simulink model "full_passive_1"  (Simulink 4.00)
settings: Solver=ode45  StartTime=0.0  StopTime=10  RelTol=1e-3
libraries: simulink3 x2
settings Model: LastModifiedBy=administrator

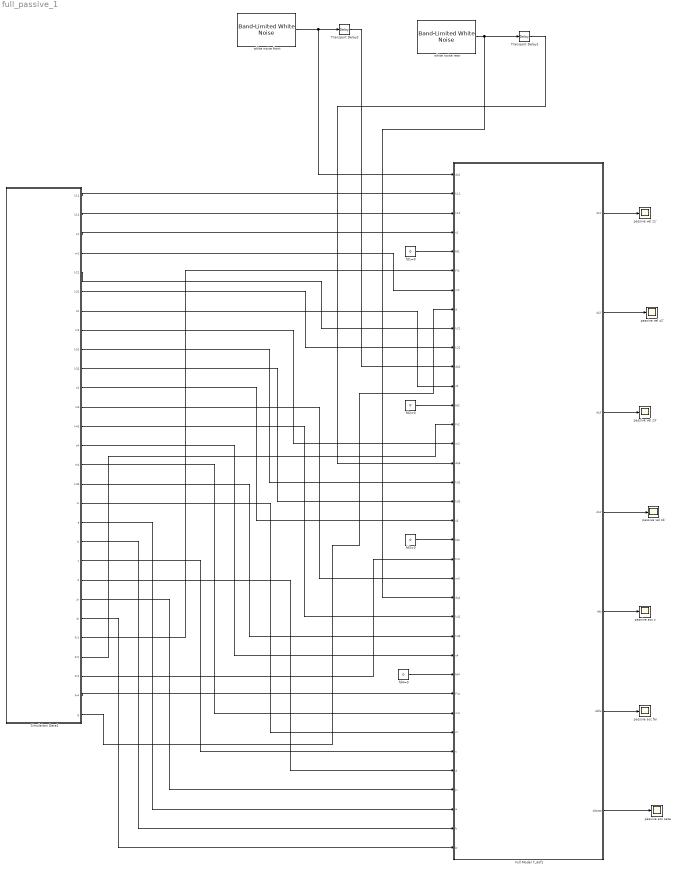
== system full_passive_1 ==
  " white noise front" : simulink3/Sources/Band-Limited White Noise  Cov=[256*10^-6]  Ts=0.01  seed=[23341]
  " white noise rear" : simulink3/Sources/Band-Limited White Noise  Cov=[256*10^-6]  Ts=0.01  seed=[23341]
  Full Model 7_dof1 : Subsystem
      settings: RTWFcnNameOpts=Auto  RTWFileNameOpts=Auto
  Simulaiton Data1 : Subsystem
      settings: RTWFcnNameOpts=Auto  RTWFileNameOpts=Auto
  Transport Delay1 : TransportDelay  DelayTime=1  InitialInput=0  BufferSize=1024  PadeOrder=0
  Transport Delay2 : TransportDelay  DelayTime=1  InitialInput=0  BufferSize=1024  PadeOrder=0
  fd1=0 : Constant  Value=0
  fd2=0 : Constant  Value=0
  fd3=0 : Constant  Value=0
  fd4=0 : Constant  Value=0
  passive acc fai : Scope
      settings: TimeRange=auto  YMin=-5  YMax=5  SaveToWorkspace=off  SaveName=ScopeData  LimitDataPoints=on  MaxDataPoints=5000
  passive acc seta : Scope
      settings: TimeRange=auto  YMin=-5  YMax=5  SaveToWorkspace=off  SaveName=ScopeData14  LimitDataPoints=on  MaxDataPoints=5000
  passive acc z : Scope
      settings: TimeRange=auto  YMin=-5  YMax=5  SaveToWorkspace=off  LimitDataPoints=on  MaxDataPoints=5000
  passive vel z1' : Scope
      settings: TimeRange=auto  YMin=-5  YMax=5  SaveToWorkspace=off  SaveName=ScopeData5  LimitDataPoints=on  MaxDataPoints=5000
  passive vel z2' : Scope
      settings: TimeRange=auto  YMin=-5  YMax=5  SaveToWorkspace=off  SaveName=ScopeData4  LimitDataPoints=on  MaxDataPoints=5000
  passive vel z3' : Scope
      settings: TimeRange=auto  YMin=-5  YMax=5  SaveToWorkspace=off  SaveName=ScopeData3  LimitDataPoints=on  MaxDataPoints=5000
  passive vel z4' : Scope
      settings: TimeRange=auto  YMin=-5  YMax=5  SaveToWorkspace=off  SaveName=ScopeData2  LimitDataPoints=on  MaxDataPoints=5000
  wires:
  " white noise front"/1 -> Transport Delay2/1, Full Model 7_dof1/1(dq1)
  Full Model 7_dof1/7(ddseta) -> passive acc seta/1
  Full Model 7_dof1/6(ddfai) -> passive acc fai/1
  Full Model 7_dof1/5(ddz) -> passive acc z/1
  Full Model 7_dof1/4(dz4') -> passive vel z4'/1
  Full Model 7_dof1/3(dz3') -> passive vel z3'/1
  Full Model 7_dof1/2(dz2') -> passive vel z2'/1
  Full Model 7_dof1/1(dz1') -> passive vel z1'/1
  Transport Delay2/1 -> Full Model 7_dof1/11(dq2)
  " white noise rear"/1 -> Transport Delay1/1, Full Model 7_dof1/23(dq4)
  Transport Delay1/1 -> Full Model 7_dof1/16(dq3)
  fd1=0/1 -> Full Model 7_dof1/5(fd1)
  fd2=0/1 -> Full Model 7_dof1/13(fd2)
  fd3=0/1 -> Full Model 7_dof1/20(fd3)
  fd4=0/1 -> Full Model 7_dof1/27(fd4)
  Simulaiton Data1/1("k11 ") -> Full Model 7_dof1/2(k11)
  Simulaiton Data1/2(k12) -> Full Model 7_dof1/3(k12)
  Simulaiton Data1/3(c1) -> Full Model 7_dof1/4(c1)
  Simulaiton Data1/4(m1) -> Full Model 7_dof1/7(m1)
  Simulaiton Data1/5(k21) -> Full Model 7_dof1/9(k21)
  Simulaiton Data1/6(k22) -> Full Model 7_dof1/10(k22)
  Simulaiton Data1/7(c2) -> Full Model 7_dof1/12(c2)
  Simulaiton Data1/8(m2) -> Full Model 7_dof1/15(m2)
  Simulaiton Data1/9(k31) -> Full Model 7_dof1/17(k31)
  Simulaiton Data1/10(k32) -> Full Model 7_dof1/18(k32)
  Simulaiton Data1/11(c3) -> Full Model 7_dof1/19(c3)
  Simulaiton Data1/26(Fr3) -> Full Model 7_dof1/21(Fr3)
  Simulaiton Data1/12(m3) -> Full Model 7_dof1/22(m3)
  Simulaiton Data1/13(k41) -> Full Model 7_dof1/24(k41)
  Simulaiton Data1/16(k42) -> Full Model 7_dof1/25(k42)
  Simulaiton Data1/14(c4) -> Full Model 7_dof1/26(c4)
  Simulaiton Data1/27(Fr4) -> Full Model 7_dof1/28(Fr4)
  Simulaiton Data1/17(m) -> Full Model 7_dof1/30(m)
  Simulaiton Data1/15(m4) -> Full Model 7_dof1/29(m4)
  Simulaiton Data1/20(c) -> Full Model 7_dof1/31(c)
  Simulaiton Data1/21(d) -> Full Model 7_dof1/32(d)
  Simulaiton Data1/22(Jx) -> Full Model 7_dof1/33(Jx)
  Simulaiton Data1/18(a) -> Full Model 7_dof1/34(a)
  Simulaiton Data1/19(b) -> Full Model 7_dof1/35(b)
  Simulaiton Data1/23(Jy) -> Full Model 7_dof1/36(Jy)
  Simulaiton Data1/28(g) -> Full Model 7_dof1/8(g)
  Simulaiton Data1/24(Fr1) -> Full Model 7_dof1/6(Fr1)
  Simulaiton Data1/25("Fr2 ") -> Full Model 7_dof1/14(Fr2)

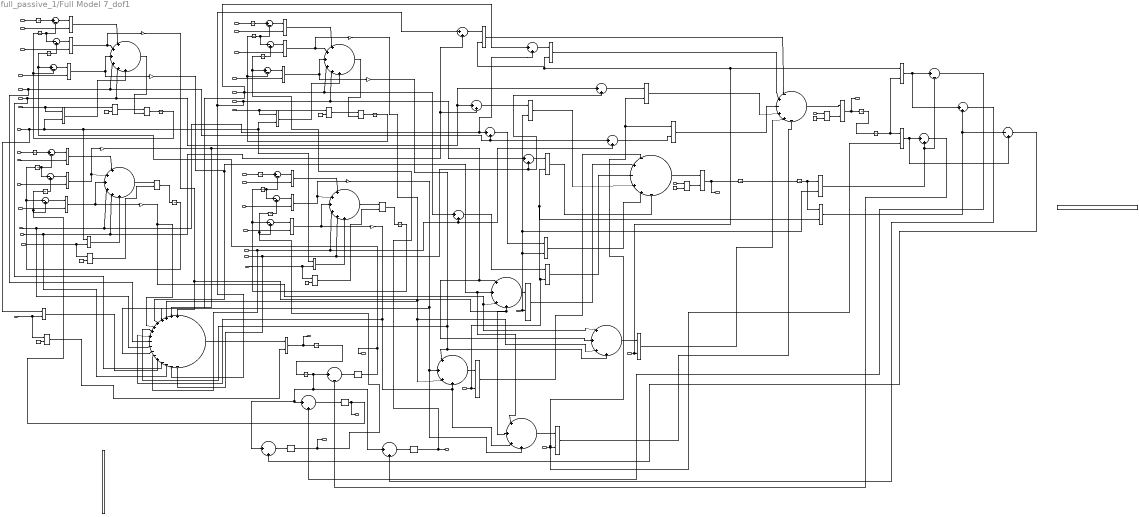
== system full_passive_1/Full Model 7_dof1 ==
  note: q1
  note: dq1
  note: z1
  note: q1-z1
  note: k11
  note: k11*(q1-z1)
  note: z1
  note: z1'
  note: k12*(z1'-z1)
  note: dz1
  note: dz1'
  note: dz1'
  note: dz1
  note: dz1'-dz1
  note: c1*(dz1'-dz1)
  note: 1/m1
  note: m1g
  note: m1ddz1
  note: ddz1
  note: dz1
  note: q2
  note: dq2
  note: q2-z2
  note: z2
  note: k21*(q2-z2)
  note: z2
  note: z2'-z2
  note: k22*(z2'-z2)
  note: z2'
  note: dz2
  note: dz2'
  note: dz2'-dz2
  note: c2*(dz2'-dz2)
  note: m2g
  note: m2ddz2
  note: 1/m2
  note: 1/m2
  note: ddz2
  note: dz2
  note: q3
  note: dq3
  note: z3
  note: q3-z3
  note: k31
  note: k31*(q3-z3)
  note: z3
  note: z3'
  note: k32*(z3'-z3)
  note: dz3
  note: dz3'
  note: dz3'
  note: dz3
  note: dz3'-dz3
  note: c3*(dz3'-dz3)
  note: 1/m3
  note: m3g
  note: m3ddz3
  note: ddz3
  note: dz3
  note: q4
  note: dq4
  note: q4-z4
  note: z4
  note: k41*(q4-z4)
  note: z4
  note: z4'-z4
  note: k42*(z4'-z4)
  note: z4'
  note: dz4
  note: dz4'
  note: dz4'-dz4
  note: c4*(dz4'-dz4)
  note: m4g
  note: m4ddz4
  note: 1/m4
  note: 1/m4
  note: ddz4
  note: dz4
  note: k12*(z1-z1')
  note: k12*(z1-z1')
  note: k22*(z2-z2')
  note: k22*(z2-z2')
  note: k32*(z3-z3')
  note: k32*(z3-z3')
  note: k42*(z4-z4')
  note: c4*(dz4-dz4')
  note: c4*(dz4-dz4')
  note: c2*(dz2-dz2')
  note: c2*(dz2'-dz2)
  note: c3*(dz3-dz3')
  note: c3*(dz3-dz3')
  note: c1*(dz1-dz1')
  note: c1*(dz1-dz1')
  note: Fr1
  note: fd1
  note: Fr2
  note: fd2
  note: fd3
  note: Fr3
  note: Fr4
  note: fd4
  note: mg
  note: mddz
  note: 1/m
  note: ddz
  note: k32*(z3-z3')
  note: c3*(dz3-dz3')
  note: k42*(z4-z4')
  note: k42*(z4-z4')
  note: c2*(dz2-dz2')
  note: k12*(z1-z1')
  note: c1*(dz1-dz1')
  note: k22*(z2-z2')
  note: Jxddfai
  note: 1/Jx
  note: ddfai
  note: k12*(z1-z1')
  note: c1*(dz1-dz1')
  note: c4*(dz4-dz4')
  note: k42*(z4-z4')
  note: -
  note: k22*(z2-z2')
  note: c2*(dz2-dz2')
  note: k32*(z3-z3')
  note: c3*(dz3-dz3')
  note: +
  note: fd1
  note: fd4
  note: -
  note: Fr1
  note: Fr4
  note: +
  note: fd2
  note: fd3
  note: +
  note: Fr2
  note: -
  note: Jyddseta
  note: 1/Jy
  note: ddseta
  note: dz
  note: z
  note: dseta
  note: seta
  note: dfai
  note: fai
  note: a
  note: a*seta
  note: d
  note: d*fai
  note: z1'
  note: d*fai
  note: dz1'
  note: b
  note: seta
  note: b*seta
  note: b*seta-d*fai
  note: z2'
  note: dz2'
  note: c*fai
  note: b*seta+c*fai
  note: z3'
  note: dz3'
  note: c*fai
  note: a*seta-c*fai
  note: z4'
  note: dz4'
  dq1 : Inport  Port=1  LatchInput=off
  k11 : Inport  Port=2  LatchInput=off
  k12 : Inport  Port=3  LatchInput=off
  c1 : Inport  Port=4  LatchInput=off
  fd1 : Inport  Port=5  LatchInput=off
  Fr1 : Inport  Port=6  LatchInput=off
  m1 : Inport  Port=7  LatchInput=off
  g : Inport  Port=8  LatchInput=off
  k21 : Inport  Port=9  LatchInput=off
  k22 : Inport  Port=10  LatchInput=off
  dq2 : Inport  Port=11  LatchInput=off
  c2 : Inport  Port=12  LatchInput=off
  fd2 : Inport  Port=13  LatchInput=off
  Fr2 : Inport  Port=14  LatchInput=off
  m2 : Inport  Port=15  LatchInput=off
  dq3 : Inport  Port=16  LatchInput=off
  k31 : Inport  Port=17  LatchInput=off
  k32 : Inport  Port=18  LatchInput=off
  c3 : Inport  Port=19  LatchInput=off
  fd3 : Inport  Port=20  LatchInput=off
  Fr3 : Inport  Port=21  LatchInput=off
  m3 : Inport  Port=22  LatchInput=off
  dq4 : Inport  Port=23  LatchInput=off
  k41 : Inport  Port=24  LatchInput=off
  k42 : Inport  Port=25  LatchInput=off
  c4 : Inport  Port=26  LatchInput=off
  fd4 : Inport  Port=27  LatchInput=off
  Fr4 : Inport  Port=28  LatchInput=off
  m4 : Inport  Port=29  LatchInput=off
  m : Inport  Port=30  LatchInput=off
  c : Inport  Port=31  LatchInput=off
  d : Inport  Port=32  LatchInput=off
  Jx : Inport  Port=33  LatchInput=off
  a : Inport  Port=34  LatchInput=off
  b : Inport  Port=35  LatchInput=off
  Jy : Inport  Port=36  LatchInput=off
  " " : Integrator  ExternalReset=none  InitialConditionSource=internal  InitialCondition=0  LimitOutput=off  UpperSaturationLimit=inf  LowerSaturationLimit=-inf  ShowSaturationPort=off  ShowStatePort=off  AbsoluteTolerance=auto
  "  " : Integrator  ExternalReset=none  InitialConditionSource=internal  InitialCondition=0  LimitOutput=off  UpperSaturationLimit=inf  LowerSaturationLimit=-inf  ShowSaturationPort=off  ShowStatePort=off  AbsoluteTolerance=auto
  Constant{,1..6} (7 alike) : Constant  Value=-1
  Derivative{,1..3} (4 alike) : Derivative
  Gain{,1..7} (8 alike) : Gain  Gain=-1  Multiplication=Element-wise(K.*u)  SaturateOnIntegerOverflow=on
  Integrator{,1..11} (12 alike) : Integrator  ExternalReset=none  InitialConditionSource=internal  InitialCondition=0  LimitOutput=off  UpperSaturationLimit=inf  LowerSaturationLimit=-inf  ShowSaturationPort=off  ShowStatePort=off  AbsoluteTolerance=auto
  Integrator for  dq{1..5,7..9} (8 alike) : Integrator  ExternalReset=none  InitialConditionSource=internal  InitialCondition=0  LimitOutput=off  UpperSaturationLimit=inf  LowerSaturationLimit=-inf  ShowSaturationPort=off  ShowStatePort=off  AbsoluteTolerance=auto
  Math Function{,1..6} (7 alike) : Math  Operator=pow  OutputSignalType=auto
  Product{,1..41} (42 alike) : Product  Inputs=2  Multiplication=Element-wise(.*)  SaturateOnIntegerOverflow=on
  Sum{,2,4,8,10,12,32..33} (8 alike) : Sum  Inputs=|+-  SaturateOnIntegerOverflow=on
  Sum{1,5..6,9,13..14,37} (7 alike) : Sum  Inputs=|-+  SaturateOnIntegerOverflow=on
  Sum{3,7,11,15} (4 alike) : Sum  Inputs=|++++++  SaturateOnIntegerOverflow=on
  Sum16 : Sum  Inputs=++++++++----+----  SaturateOnIntegerOverflow=on
  Sum{17..18,24..25} (4 alike) : Sum  Inputs=|++++  SaturateOnIntegerOverflow=on
  Sum{19..22,26..29,31,34..36,38} (13 alike) : Sum  Inputs=|++  SaturateOnIntegerOverflow=on
  Sum23 : Sum  Inputs=|-+-++-  SaturateOnIntegerOverflow=on
  Sum30 : Sum  Inputs=|-+-++-  SaturateOnIntegerOverflow=on
  dz1' : Outport  Port=1
  dz2' : Outport  Port=2
  dz3' : Outport  Port=3
  dz4' : Outport  Port=4
  ddz : Outport  Port=5
  ddfai : Outport  Port=6
  ddseta : Outport  Port=7
  wires:
  Integrator for  dq1/1 -> Sum/1
  dq1/1 -> Integrator for  dq1/1
  Integrator/1 -> Sum/2, Sum1/1
  Sum/1 -> Product/1
  k11/1 -> Product/2
  Product/1 -> Sum3/1
  Integrator1/1 -> Sum1/2
  Sum1/1 -> Product1/1
  k12/1 -> Product1/2
  Product1/1 -> Sum3/2, Gain/1
  c1/1 -> Product3/2
  Sum2/1 -> Product3/1
  Product3/1 -> Sum3/3, Gain7/1
  fd1/1 -> Sum16/9, Sum20/2, Sum26/1, Sum3/4
  Fr1/1 -> Sum16/14, Sum22/1, Sum27/1, Sum3/5
  m1/1 -> Math Function/1, Product4/1
  g/1 -> Product4/2, Product9/1, Product16/2, Product21/1, Product22/1
  Constant/1 -> Math Function/2
  Math Function/1 -> Product10/1
  Product4/1 -> Sum3/6
  Sum3/1 -> Product10/2
  Product10/1 -> Integrator2/1
  Integrator2/1 -> Sum2/2, Integrator/1
  Integrator for  dq2/1 -> Sum4/1
  dq2/1 -> Integrator for  dq2/1
  Sum4/1 -> Product6/1
  Integrator for  dq3/1 -> Sum4/2, Sum5/1
  k21/1 -> Product6/2
  Product6/1 -> Sum7/1
  Integrator for  dq4/1 -> Sum5/2
  Sum5/1 -> Product7/1
  k22/1 -> Product7/2
  Product7/1 -> Sum7/2, Gain1/1
  c2/1 -> Product8/2
  Sum6/1 -> Product8/1
  Product8/1 -> Sum7/3, Gain5/1
  fd2/1 -> Sum16/10, Sum7/4, Sum20/1, Sum28/2
  Fr2/1 -> Sum16/15, Sum7/5, Sum22/2, Sum29/2
  Product9/1 -> Sum7/6
  m2/1 -> Product9/2, Math Function1/1
  Sum7/1 -> Product11/1
  Constant1/1 -> Math Function1/2
  Math Function1/1 -> Product11/2
  Product11/1 -> Integrator for  dq5/1
  Integrator for  dq5/1 -> Integrator for  dq3/1, Sum6/1
  " "/1 -> Sum8/1
  dq3/1 -> " "/1
  Integrator3/1 -> Sum8/2, Sum9/1
  Sum8/1 -> Product12/1
  k31/1 -> Product12/2
  Product12/1 -> Sum11/1
  Integrator4/1 -> Sum9/2
  Sum9/1 -> Product13/1
  k32/1 -> Product13/2
  Product13/1 -> Sum11/2, Gain2/1
  c3/1 -> Product15/2
  Sum10/1 -> Product15/1
  Product15/1 -> Sum11/3, Gain6/1
  fd3/1 -> Sum16/11, Sum11/4, Sum19/1, Sum28/1
  Fr3/1 -> Sum11/5, Sum21/1, Sum16/16, Sum29/1
  m3/1 -> Math Function2/1, Product16/1
  Constant2/1 -> Math Function2/2
  Math Function2/1 -> Product14/1
  Product16/1 -> Sum11/6
  Sum11/1 -> Product14/2
  Product14/1 -> Integrator5/1
  Integrator5/1 -> Sum10/2, Integrator3/1
  "  "/1 -> Sum12/1
  dq4/1 -> "  "/1
  Sum12/1 -> Product18/1
  Integrator for  dq7/1 -> Sum12/2, Sum13/1
  k41/1 -> Product18/2
  Product18/1 -> Sum15/1
  Integrator for  dq8/1 -> Sum13/2
  Sum13/1 -> Product19/1
  k42/1 -> Product19/2
  Product19/1 -> Sum15/2, Gain3/1
  c4/1 -> Product20/2
  Sum14/1 -> Product20/1
  Product20/1 -> Sum15/3, Gain4/1
  fd4/1 -> Sum16/12, Sum15/4, Sum19/2, Sum26/2
  Fr4/1 -> Sum16/17, Sum15/5, Sum21/2, Sum27/2
  Product21/1 -> Sum15/6
  m4/1 -> Product21/2, Math Function3/1
  Sum15/1 -> Product17/1
  Constant3/1 -> Math Function3/2
  Math Function3/1 -> Product17/2
  Product17/1 -> Integrator for  dq9/1
  Integrator for  dq9/1 -> Integrator for  dq7/1, Sum14/1
  Gain/1 -> Sum16/1, Sum18/4, Sum24/2
  Gain1/1 -> Sum16/2, Sum18/1, Sum25/2
  Gain2/1 -> Sum16/3, Sum17/3, Sum25/3
  Gain3/1 -> Sum16/4, Sum17/2, Sum24/4
  Gain4/1 -> Sum16/8, Sum17/4, Sum24/3
  Gain5/1 -> Sum16/6, Sum18/3, Sum25/1
  Gain6/1 -> Sum16/7, Sum17/1, Sum25/4
  Gain7/1 -> Sum16/5, Sum18/2, Sum24/1
  m/1 -> Product22/2, Math Function4/1
  Product22/1 -> Sum16/13
  Sum16/1 -> Product23/1
  Constant4/1 -> Math Function4/2
  Math Function4/1 -> Product23/2
  Product23/1 -> Integrator6/1, ddz/1
  Sum17/1 -> Product24/1
  c/1 -> Product24/2, Product26/2, Product28/2, Product41/2
  Product24/1 -> Sum23/1
  Sum18/1 -> Product25/1
  d/1 -> Product25/2, Product27/2, Product29/2, Product39/2
  Product25/1 -> Sum23/2
  Sum19/1 -> Product26/1
  Product26/1 -> Sum23/3
  Sum20/1 -> Product27/1
  Sum21/1 -> Product28/1
  Sum22/1 -> Product29/1
  Product29/1 -> Sum23/4
  Product27/1 -> Sum23/5
  Product28/1 -> Sum23/6
  Sum23/1 -> Product30/1
  Jx/1 -> Math Function5/1
  Constant5/1 -> Math Function5/2
  Math Function5/1 -> Product30/2
  Product30/1 -> Integrator10/1, ddfai/1
  Sum24/1 -> Product31/1
  a/1 -> Product31/2, Product33/1, Product34/2, Product38/2
  Product31/1 -> Sum30/6
  Sum25/1 -> Product32/1
  b/1 -> Product32/2, Product40/1, Product35/2, Product36/2
  Product32/1 -> Sum30/5
  Sum26/1 -> Product33/2
  Product33/1 -> Sum30/3
  Sum27/1 -> Product34/1
  Product34/1 -> Sum30/4
  Sum28/1 -> Product35/1
  Product35/1 -> Sum30/2
  Sum29/1 -> Product36/1
  Product36/1 -> Sum30/1
  Sum30/1 -> Product37/1
  Jy/1 -> Math Function6/1
  Constant6/1 -> Math Function6/2
  Math Function6/1 -> Product37/2
  Product37/1 -> Integrator8/1, ddseta/1
  Integrator6/1 -> Integrator7/1
  Integrator7/1 -> Sum36/1, Sum34/1, Sum38/1, Sum32/1
  Integrator8/1 -> Integrator9/1
  Integrator9/1 -> Product38/1, Product40/2
  Integrator10/1 -> Integrator11/1
  Integrator11/1 -> Product39/1, Product41/1
  Product38/1 -> Sum31/1, Sum37/2
  Product39/1 -> Sum31/2, Sum33/2
  Sum31/1 -> Sum32/2
  Sum32/1 -> Derivative/1
  Derivative/1 -> Sum2/1, Integrator1/1, dz1'/1
  Product40/1 -> Sum33/1, Sum35/1
  Sum33/1 -> Sum34/2
  Sum34/1 -> Derivative1/1
  Derivative1/1 -> Integrator for  dq4/1, Sum6/2, dz2'/1
  Product41/1 -> Sum35/2, Sum37/1
  Sum35/1 -> Sum36/2
  Sum36/1 -> Derivative2/1
  Derivative2/1 -> Integrator4/1, Sum10/1, dz3'/1
  Sum37/1 -> Sum38/2
  Sum38/1 -> Derivative3/1
  Derivative3/1 -> Integrator for  dq8/1, Sum14/2, dz4'/1

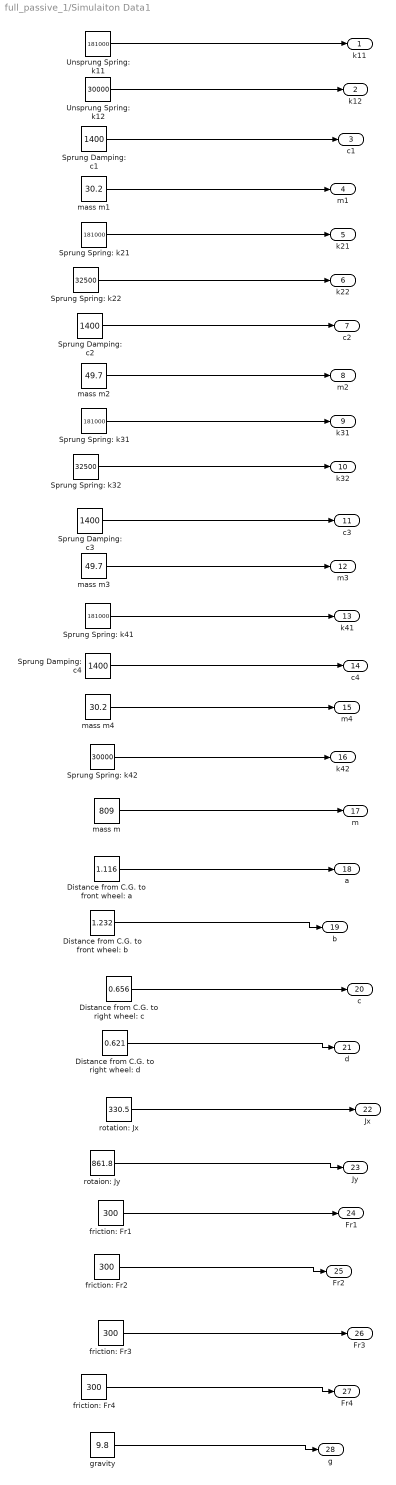
== system full_passive_1/Simulaiton Data1 ==
   Sprung Damping: c{1..4} (4 alike) : Constant  Value=1400
  " Sprung Spring: k21" : Constant  Value=181000
  " Sprung Spring: k22" : Constant  Value=32500
  " Sprung Spring: k31" : Constant  Value=181000
  " Sprung Spring: k32" : Constant  Value=32500
  " Sprung Spring: k41" : Constant  Value=181000
  " Sprung Spring: k42" : Constant  Value=30000
  Distance from C.G. to front wheel: a : Constant  Value=1.116
  Distance from C.G. to front wheel: b : Constant  Value=1.232
  Distance from C.G. to right wheel: c : Constant  Value=0.656
  Distance from C.G. to right wheel: d : Constant  Value=0.621
  Unsprung Spring: k11 : Constant  Value=181000
  Unsprung Spring: k12 : Constant  Value=30000
  friction: Fr{1..4} (4 alike) : Constant  Value=300
  gravity : Constant  Value=9.8
  mass m : Constant  Value=809
  mass m1 : Constant  Value=30.2
  mass m2 : Constant  Value=49.7
  mass m3 : Constant  Value=49.7
  mass m4 : Constant  Value=30.2
  rotaion: Jy : Constant  Value=861.8
  rotation: Jx : Constant  Value=330.5
  "k11 " : Outport  Port=1
  k12 : Outport  Port=2
  c1 : Outport  Port=3
  m1 : Outport  Port=4
  k21 : Outport  Port=5
  k22 : Outport  Port=6
  c2 : Outport  Port=7
  m2 : Outport  Port=8
  k31 : Outport  Port=9
  k32 : Outport  Port=10
  c3 : Outport  Port=11
  m3 : Outport  Port=12
  k41 : Outport  Port=13
  c4 : Outport  Port=14
  m4 : Outport  Port=15
  k42 : Outport  Port=16
  m : Outport  Port=17
  a : Outport  Port=18
  b : Outport  Port=19
  c : Outport  Port=20
  d : Outport  Port=21
  Jx : Outport  Port=22
  Jy : Outport  Port=23
  Fr1 : Outport  Port=24
  "Fr2 " : Outport  Port=25
  Fr3 : Outport  Port=26
  Fr4 : Outport  Port=27
  g : Outport  Port=28
  wires:
  Unsprung Spring: k11/1 -> "k11 "/1
  " Sprung Damping: c1"/1 -> c1/1
  " Sprung Damping: c2"/1 -> c2/1
  Distance from C.G. to front wheel: a/1 -> a/1
  " Sprung Spring: k21"/1 -> k21/1
  Unsprung Spring: k12/1 -> k12/1
  " Sprung Spring: k22"/1 -> k22/1
  mass m1/1 -> m1/1
  mass m2/1 -> m2/1
  " Sprung Spring: k31"/1 -> k31/1
  " Sprung Spring: k32"/1 -> k32/1
  " Sprung Damping: c3"/1 -> c3/1
  mass m3/1 -> m3/1
  " Sprung Spring: k41"/1 -> k41/1
  " Sprung Damping: c4"/1 -> c4/1
  mass m4/1 -> m4/1
  " Sprung Spring: k42"/1 -> k42/1
  mass m/1 -> m/1
  Distance from C.G. to front wheel: b/1 -> b/1
  Distance from C.G. to right wheel: c/1 -> c/1
  Distance from C.G. to right wheel: d/1 -> d/1
  rotation: Jx/1 -> Jx/1
  rotaion: Jy/1 -> Jy/1
  friction: Fr1/1 -> Fr1/1
  friction: Fr2/1 -> "Fr2 "/1
  friction: Fr3/1 -> Fr3/1
  friction: Fr4/1 -> Fr4/1
  gravity/1 -> g/1
